simulink model "Schedule_generator"  (R2018b)
settings: Solver=VariableStepAuto  StartTime=0.0  StopTime=n_T  RelTol=1e-3
undefined symbols (not defined in the file or in its folder): n_AT, n_pre, n_T
libraries: dspswit3 x5
settings Model: Creator=Jorrit de Jong  LastModifiedBy=Jorrit de Jong

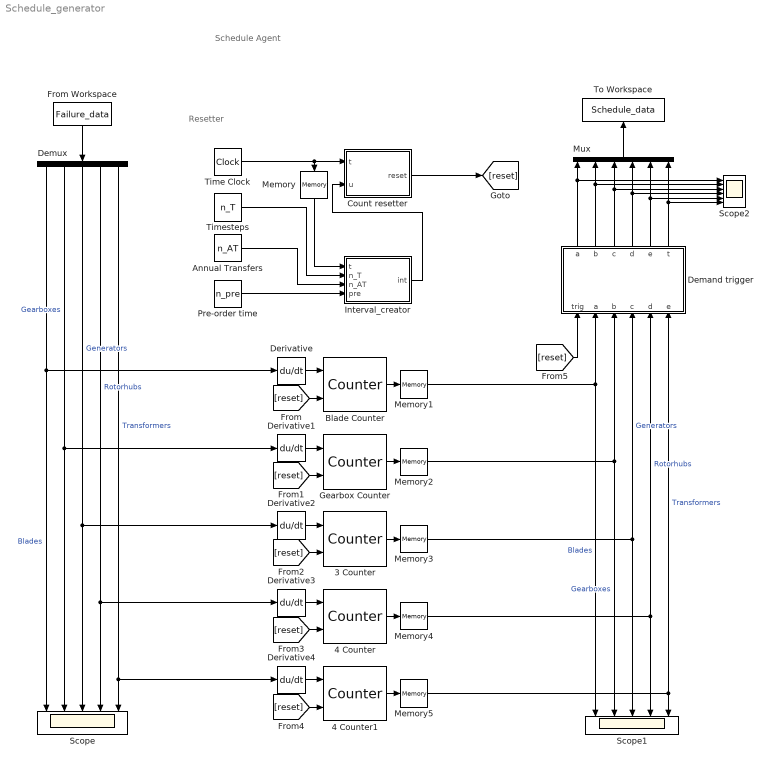
== system Schedule_generator ==
  note: Resetter
  note: Schedule Agent
  3 Counter : dspswit3/Counter  Direction=Up  CountEvent=Rising edge  CounterSize=User defined  MaxCount=255  InitialCount=0  Output=Count  HitValue=32  ResetInput=on  SamplesPerFrame=1  Ts=1  CntDtype=double  HitDtype=Logical
  4 Counter : dspswit3/Counter  Direction=Up  CountEvent=Rising edge  CounterSize=User defined  MaxCount=255  InitialCount=0  Output=Count  HitValue=32  ResetInput=on  SamplesPerFrame=1  Ts=1  CntDtype=double  HitDtype=Logical
  4 Counter1 : dspswit3/Counter  Direction=Up  CountEvent=Rising edge  CounterSize=User defined  MaxCount=255  InitialCount=0  Output=Count  HitValue=32  ResetInput=on  SamplesPerFrame=1  Ts=1  CntDtype=double  HitDtype=Logical
  Annual Transfers : Constant  Value=n_AT
  Blade Counter : dspswit3/Counter  Direction=Up  CountEvent=Rising edge  CounterSize=User defined  MaxCount=255  InitialCount=0  Output=Count  HitValue=32  ResetInput=on  SamplesPerFrame=1  Ts=1  CntDtype=double  HitDtype=Logical
  Count resetter : MATLAB Function  TreatAsAtomicUnit=on
  Demand trigger : MATLAB Function  TreatAsAtomicUnit=on
  Demux : Demux  Outputs=5
  Derivative{,1..4} (5 alike) : Derivative
  From Workspace : FromWorkspace  VariableName=Failure_data  SampleTime=0
  Gearbox Counter : dspswit3/Counter  Direction=Up  CountEvent=Rising edge  CounterSize=User defined  MaxCount=255  InitialCount=0  Output=Count  HitValue=32  ResetInput=on  SamplesPerFrame=1  Ts=1  CntDtype=double  HitDtype=Logical
  Interval_creator : MATLAB Function  TreatAsAtomicUnit=on
  Memory{,1..5} (6 alike) : Memory
  Mux : Mux  Inputs=6
  Pre-order time : Constant  Value=n_pre
  Scope : Scope  NumInputPorts=5
  Scope1 : Scope  NumInputPorts=5
  Scope2 : Scope  NumInputPorts=6
  Time Clock : DigitalClock
  Timesteps : Constant  Value=n_T
  To Workspace : ToWorkspace  VariableName=Schedule_data  SaveFormat=Timeseries  SampleTime=1
  wires:
  Demux/1 -> Scope/1, Derivative/1  "Blades"
  Demux/2 -> Scope/2, Derivative1/1  "Gearboxes"
  Demux/3 -> Scope/3, Derivative2/1  "Generators"
  Demux/4 -> Derivative3/1, Scope/4  "Rotorhubs"
  Demux/5 -> Derivative4/1, Scope/5  "Transformers"
  Annual Transfers/1 -> Interval_creator/3(n_AT)
  Timesteps/1 -> Interval_creator/2(n_T)
  Time Clock/1 -> Count resetter/1(t), Memory/1
  Interval_creator/1(int) -> Count resetter/2(u)
  Memory/1 -> Interval_creator/1(t)
  Blade Counter/1 -> Memory1/1
  Derivative/1 -> Blade Counter/1
  Derivative1/1 -> Gearbox Counter/1
  Count resetter/1(reset) -> [reset]
  [reset] -> Blade Counter/2
  [reset] -> Gearbox Counter/2
  Gearbox Counter/1 -> Memory2/1
  Memory1/1 -> Demand trigger/2("a "), Scope1/1  "Blades"
  Memory2/1 -> Demand trigger/3("b "), Scope1/2  "Gearboxes"
  [reset] -> 3 Counter/2
  Memory3/1 -> Demand trigger/4("c "), Scope1/3  "Generators"
  Derivative2/1 -> 3 Counter/1
  3 Counter/1 -> Memory3/1
  4 Counter/1 -> Memory4/1
  Memory4/1 -> Demand trigger/5("d "), Scope1/4  "Rotorhubs"
  Derivative3/1 -> 4 Counter/1
  [reset] -> 4 Counter/2
  [reset] -> 4 Counter1/2
  Memory5/1 -> Demand trigger/6("e "), Scope1/5  "Transformers"
  Derivative4/1 -> 4 Counter1/1
  4 Counter1/1 -> Memory5/1
  Pre-order time/1 -> Interval_creator/4(pre)
  Demand trigger/1(a) -> Scope2/1, Mux/1
  Demand trigger/2(b) -> Scope2/2, Mux/2
  Demand trigger/3(c) -> Scope2/3, Mux/3
  Demand trigger/4(d) -> Scope2/4, Mux/4
  Demand trigger/5(e) -> Scope2/5, Mux/5
  Mux/1 -> To Workspace/1
  [reset] -> Demand trigger/1(trig)
  From Workspace/1 -> Demux/1
  Demand trigger/6(t) -> Mux/6, Scope2/6

== matlab function Schedule_generator/Interval_creator ==
  data: t input; n_T input; n_AT input; int output; pre input
function int = fcn(t,n_T,n_AT,pre)

int = ((n_T/n_AT)*fix(t/(n_T/n_AT))+(n_T/n_AT))-pre;


% u = (n_T/n_AT)

== matlab function Schedule_generator/Count resetter ==
  data: t input; u input; reset output
function reset  = fcn(t,u)
if t == u
    %y = f;
    reset = 1; 
else
    %y = 0;
    reset = 0;
end

== matlab function Schedule_generator/Demand trigger ==
  data: trig input; a output; a input; b input; c input; d input; e input; b output; c output; d output; e output; t output
function [a,b,c,d,e,t] = fcn(trig,a,b,c,d,e)
if trig == 1;
    a = a;
    b = b;
    c = c;
    d = d;
    e = e;
    t = a + b + c + d + e;
else
    a = 0;
    b = 0;
    c = 0;
    d = 0;
    e = 0;
    t = 0;
end
